simulink model "sampleModel100"  (R2021b)
settings: Solver=VariableStepAuto  StartTime=0.0  StopTime=10.0  RelTol=1e-3
undefined symbols (not defined in the file or in its folder): DiscIntNeverNeededParam, magnitude, Newton, Raphson
libraries: simulink x6
settings Model: Creator=user  LastModifiedBy=user

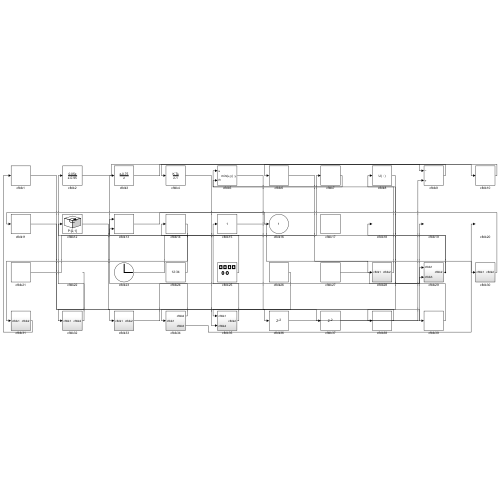
[thumbnail: Simulink's stored preview of the top-level diagram]
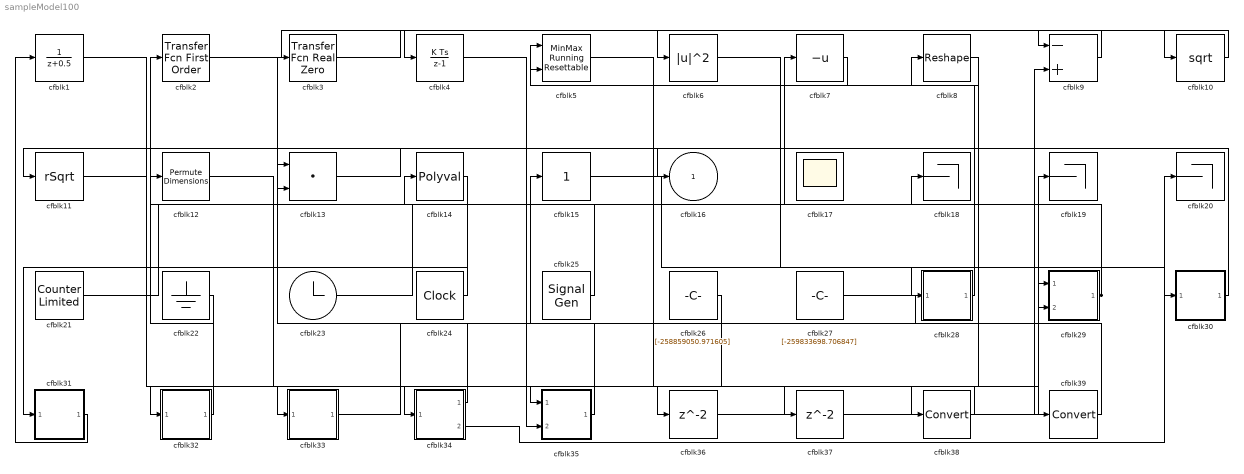
== system sampleModel100 ==
  cfblk1 : DiscreteTransferFcn  SampleTime=1
  cfblk10 : Sqrt  SaturateOnIntegerOverflow=on
  cfblk11 : Sqrt  Operator=rSqrt  AlgorithmType=Newton-Raphson  SaturateOnIntegerOverflow=on
  cfblk12 : PermuteDimensions
  cfblk13 : DotProduct  InputSameDT=on  OutDataTypeStr=Inherit: Inherit via internal rule
  cfblk14 : Polyval  Coefs=[ +2.081618890e-019, -1.441693666e-014, +4.719686976e-010, -8.536869453e-006, +1.621573104e-001, -8.087801117e+001 ]
  cfblk15 : simulink/Math Operations/Slider Gain  gain=1  low=0  high=2
  cfblk17 : Scope
      settings: Floating=on
  cfblk18 : Terminator
  cfblk19 : Terminator
  cfblk2 : simulink/Discrete/Transfer Fcn First Order  PoleZ=0.95  ICPrevOutput=0.0  DoSatur=off
  cfblk20 : Terminator
  cfblk21 : simulink/Sources/Counter Limited  uplimit=[247.000000]  tsamp=-1
  cfblk22 : Ground
  cfblk23 : Clock
  cfblk24 : DigitalClock
  cfblk25 : SignalGenerator  WaveForm=square  Amplitude=[720675936.087589]
  cfblk26 : Constant  Value=[-258859050.971605]  SampleTime=1
  cfblk27 : Constant  Value=[-259833698.706847]  SampleTime=1
  cfblk28 : Subsystem
  cfblk29 : Subsystem
  cfblk3 : simulink/Discrete/Transfer Fcn Real Zero  ZeroZ=0.75  ICPrevInput=0.0  DoSatur=off
      settings: SourceProductBaseCode=SL
  cfblk30 : Subsystem
  cfblk31 : Subsystem
  cfblk32 : Subsystem
  cfblk33 : Subsystem
  cfblk34 : Subsystem
  cfblk35 : Subsystem
  cfblk36 : Delay  SampleTime=1
  cfblk37 : Delay  SampleTime=1
  cfblk38 : DataTypeConversion
  cfblk39 : DataTypeConversion
  cfblk4 : DiscreteIntegrator  ICPrevOutput=DiscIntNeverNeededParam  ICPrevScaledInput=DiscIntNeverNeededParam
  cfblk5 : simulink/Math Operations/MinMax Running Resettable  Function=min  vinit=0.0
  cfblk6 : Math  Operator=magnitude^2  SaturateOnIntegerOverflow=on
  cfblk7 : UnaryMinus
  cfblk8 : Reshape
  cfblk9 : Sum  Inputs=-+
  cfblk16 : Outport
  wires:
  cfblk14/1 -> cfblk31/1(cfblk1)
  cfblk30/1(cfblk2) -> cfblk11/1
  cfblk2/1 -> cfblk9/1
  cfblk23/1 -> cfblk7/1
  cfblk24/1 -> cfblk3/1
  cfblk28/1(cfblk2) -> cfblk5/1
  cfblk27/1 -> cfblk19/1
  cfblk7/1 -> cfblk5/2
  cfblk22/1 -> cfblk32/1(cfblk1)
  cfblk32/1(cfblk2) -> cfblk2/1
  cfblk15/1 -> cfblk28/1(cfblk1)
  cfblk31/1(cfblk2) -> cfblk1/1
  cfblk26/1 -> cfblk35/1(cfblk1)
  cfblk29/1(cfblk2) -> cfblk12/1, cfblk18/1
  cfblk4/1 -> cfblk35/2(cfblk4)
  cfblk9/1 -> cfblk4/1
  cfblk21/1 -> cfblk13/1
  cfblk25/1 -> cfblk14/1
  cfblk35/1(cfblk2) -> cfblk15/1
  cfblk13/1 -> cfblk16/1
  cfblk33/1(cfblk2) -> cfblk29/1(cfblk1)
  cfblk1/1 -> cfblk33/1(cfblk1)
  cfblk34/1(cfblk2) -> cfblk13/2
  cfblk3/1 -> cfblk10/1
  cfblk34/2(cfblk3) -> cfblk20/1
  cfblk10/1 -> cfblk6/1
  cfblk6/1 -> cfblk30/1(cfblk1)
  cfblk12/1 -> cfblk36/1
  cfblk36/1 -> cfblk29/2(cfblk3)
  cfblk5/1 -> cfblk37/1
  cfblk37/1 -> cfblk9/2
  cfblk8/1 -> cfblk38/1
  cfblk38/1 -> cfblk34/1(cfblk1)
  cfblk11/1 -> cfblk39/1
  cfblk39/1 -> cfblk8/1

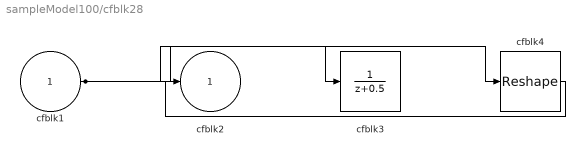
== system sampleModel100/cfblk28 ==
  cfblk1 : Inport
  cfblk3 : DiscreteTransferFcn  SampleTime=1
  cfblk4 : Reshape
  cfblk2 : Outport
  wires:
  cfblk1/1 -> cfblk4/1, cfblk3/1
  cfblk4/1 -> cfblk2/1

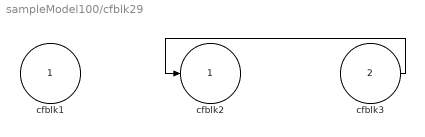
== system sampleModel100/cfblk29 ==
  cfblk1 : Inport
  cfblk3 : Inport  Port=2
  cfblk2 : Outport
  wires:
  cfblk3/1 -> cfblk2/1

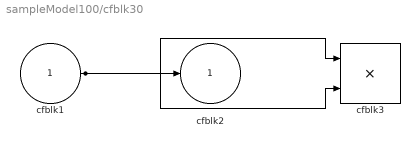
== system sampleModel100/cfblk30 ==
  cfblk1 : Inport
  cfblk3 : Product
  cfblk2 : Outport
  wires:
  cfblk1/1 -> cfblk2/1, cfblk3/1, cfblk3/2

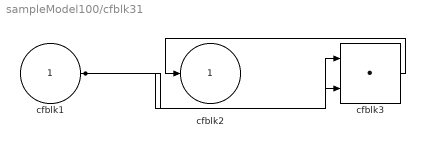
== system sampleModel100/cfblk31 ==
  cfblk1 : Inport
  cfblk3 : DotProduct  InputSameDT=on  OutDataTypeStr=Inherit: Inherit via internal rule
  cfblk2 : Outport
  wires:
  cfblk3/1 -> cfblk2/1
  cfblk1/1 -> cfblk3/1, cfblk3/2

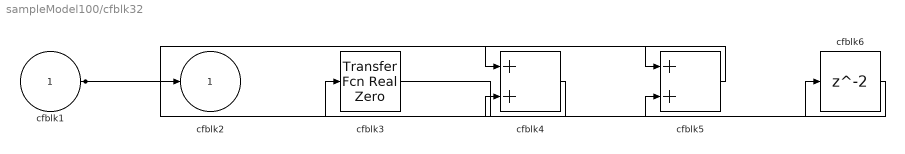
== system sampleModel100/cfblk32 ==
  cfblk1 : Inport
  cfblk3 : simulink/Discrete/Transfer Fcn Real Zero  ZeroZ=0.75  ICPrevInput=0.0  DoSatur=off
      settings: SourceProductBaseCode=SL
  cfblk4 : Sum
  cfblk5 : Sum
  cfblk6 : Delay  SampleTime=1
  cfblk2 : Outport
  wires:
  cfblk1/1 -> cfblk2/1, cfblk5/1, cfblk5/2
  cfblk5/1 -> cfblk4/1
  cfblk4/1 -> cfblk3/1
  cfblk3/1 -> cfblk6/1
  cfblk6/1 -> cfblk4/2

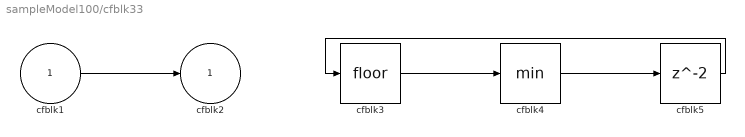
== system sampleModel100/cfblk33 ==
  cfblk1 : Inport
  cfblk3 : Rounding
  cfblk4 : MinMax
  cfblk5 : Delay  SampleTime=1
  cfblk2 : Outport
  wires:
  cfblk1/1 -> cfblk2/1
  cfblk3/1 -> cfblk4/1
  cfblk4/1 -> cfblk5/1
  cfblk5/1 -> cfblk3/1

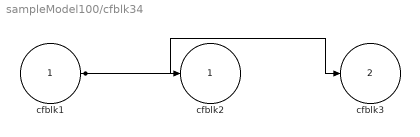
== system sampleModel100/cfblk34 ==
  cfblk1 : Inport
  cfblk2 : Outport
  cfblk3 : Outport  Port=2
  wires:
  cfblk1/1 -> cfblk3/1, cfblk2/1

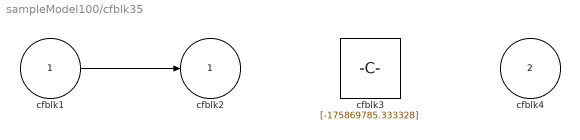
== system sampleModel100/cfblk35 ==
  cfblk1 : Inport
  cfblk4 : Inport  Port=2
  cfblk3 : Constant  Value=[-175869785.333328]  SampleTime=1
  cfblk2 : Outport
  wires:
  cfblk1/1 -> cfblk2/1
